simulink model "Switching_losses"  (R2015a)
settings: Solver=ode45  StartTime=0.0  StopTime=10.0  RelTol=1e-3
undefined symbols (not defined in the file): Vdc
settings Model: Creator=Caner  LastModifiedBy=Caner

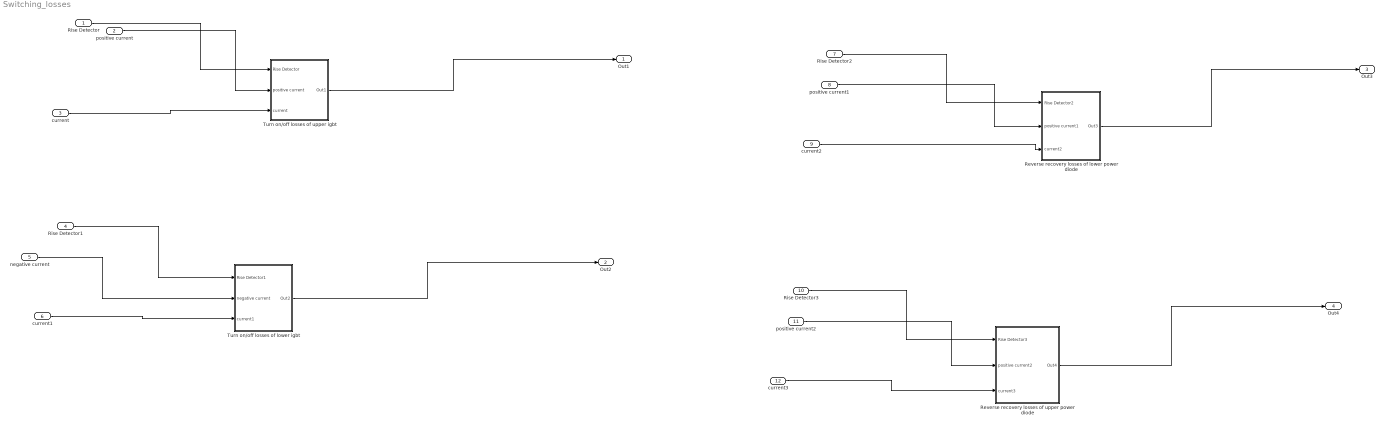
== system Switching_losses ==
  Rise Detector : Inport
  positive current : Inport  Port=2
  current : Inport  Port=3
  Rise Detector1 : Inport  Port=4
  negative current : Inport  Port=5
  current1 : Inport  Port=6
  Rise Detector2 : Inport  Port=7
  positive current1 : Inport  Port=8
  current2 : Inport  Port=9
  Rise Detector3 : Inport  Port=10
  positive current2 : Inport  Port=11
  current3 : Inport  Port=12
  "Reverse recovery losses of lower power diode " : Subsystem
  "Reverse recovery losses of upper power diode " : Subsystem
  "Turn on/off losses of lower igbt " : Subsystem
  "Turn on/off losses of upper igbt " : Subsystem
  Out1 : Outport
  Out2 : Outport  Port=2
  Out3 : Outport  Port=3
  Out4 : Outport  Port=4
  wires:
  Rise Detector/1 -> "Turn on/off losses of upper igbt "/1(Rise Detector)
  positive current/1 -> "Turn on/off losses of upper igbt "/2(positive current)
  current/1 -> "Turn on/off losses of upper igbt "/3(current)
  "Turn on/off losses of upper igbt "/1(Out1) -> Out1/1
  Rise Detector1/1 -> "Turn on/off losses of lower igbt "/1(Rise Detector1)
  negative current/1 -> "Turn on/off losses of lower igbt "/2(negative current)
  current1/1 -> "Turn on/off losses of lower igbt "/3(current1)
  "Turn on/off losses of lower igbt "/1(Out2) -> Out2/1
  Rise Detector2/1 -> "Reverse recovery losses of lower power diode "/1(Rise Detector2)
  positive current1/1 -> "Reverse recovery losses of lower power diode "/2(positive current1)
  current2/1 -> "Reverse recovery losses of lower power diode "/3(current2)
  "Reverse recovery losses of lower power diode "/1(Out3) -> Out3/1
  Rise Detector3/1 -> "Reverse recovery losses of upper power diode "/1(Rise Detector3)
  positive current2/1 -> "Reverse recovery losses of upper power diode "/2(positive current2)
  current3/1 -> "Reverse recovery losses of upper power diode "/3(current3)
  "Reverse recovery losses of upper power diode "/1(Out4) -> Out4/1

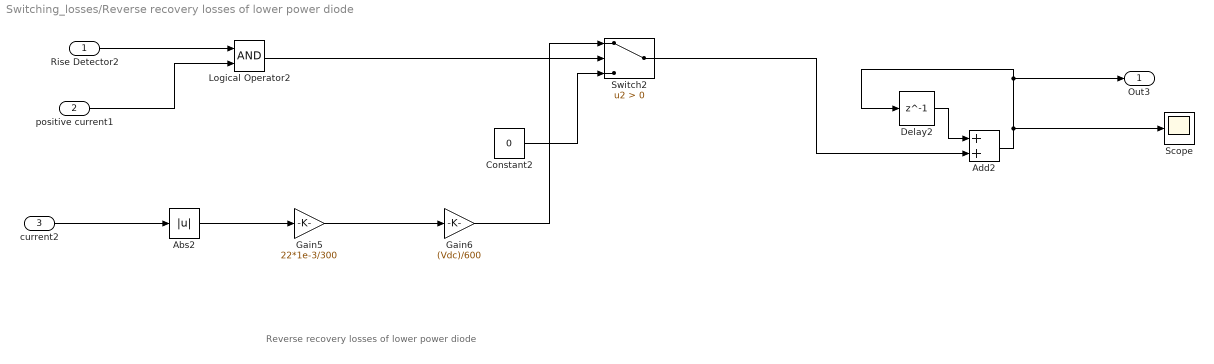
== system Switching_losses/Reverse recovery losses of lower power diode  ==
  note: Reverse recovery losses of lower power diode
  Rise Detector2 : Inport
  positive current1 : Inport  Port=2
  current2 : Inport  Port=3
  Abs2 : Abs
  Add2 : Sum
  Constant2 : Constant  Value=0
  Delay2 : Delay  DelayLength=1  InitialCondition=0
  Gain5 : Gain  Gain=22*1e-3/300
  Gain6 : Gain  Gain=(Vdc)/600
  Logical Operator2 : Logic  AllPortsSameDT=off  OutDataTypeStr=boolean
  Scope : Scope
  Switch2 : Switch  Criteria=u2 > Threshold
  Out3 : Outport
  wires:
  Gain5/1 -> Gain6/1
  Constant2/1 -> Switch2/3
  positive current1/1 -> Logical Operator2/2
  Add2/1 -> Scope/1, Out3/1, Delay2/1
  current2/1 -> Abs2/1
  Logical Operator2/1 -> Switch2/2
  Gain6/1 -> Switch2/1
  Rise Detector2/1 -> Logical Operator2/1
  Switch2/1 -> Add2/2
  Delay2/1 -> Add2/1
  Abs2/1 -> Gain5/1

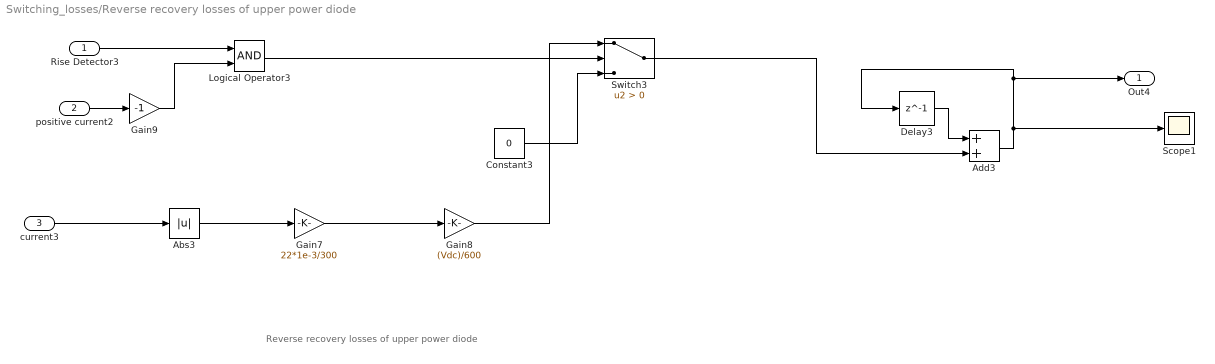
== system Switching_losses/Reverse recovery losses of upper power diode  ==
  note: Reverse recovery losses of upper power diode
  Rise Detector3 : Inport
  positive current2 : Inport  Port=2
  current3 : Inport  Port=3
  Abs3 : Abs
  Add3 : Sum
  Constant3 : Constant  Value=0
  Delay3 : Delay  DelayLength=1  InitialCondition=0
  Gain7 : Gain  Gain=22*1e-3/300
  Gain8 : Gain  Gain=(Vdc)/600
  Gain9 : Gain  Gain=-1
  Logical Operator3 : Logic  AllPortsSameDT=off  OutDataTypeStr=boolean
  Scope1 : Scope
  Switch3 : Switch  Criteria=u2 > Threshold
  Out4 : Outport
  wires:
  Abs3/1 -> Gain7/1
  Gain7/1 -> Gain8/1
  Gain8/1 -> Switch3/1
  Rise Detector3/1 -> Logical Operator3/1
  positive current2/1 -> Gain9/1
  Logical Operator3/1 -> Switch3/2
  current3/1 -> Abs3/1
  Add3/1 -> Scope1/1, Out4/1, Delay3/1
  Delay3/1 -> Add3/1
  Constant3/1 -> Switch3/3
  Gain9/1 -> Logical Operator3/2
  Switch3/1 -> Add3/2

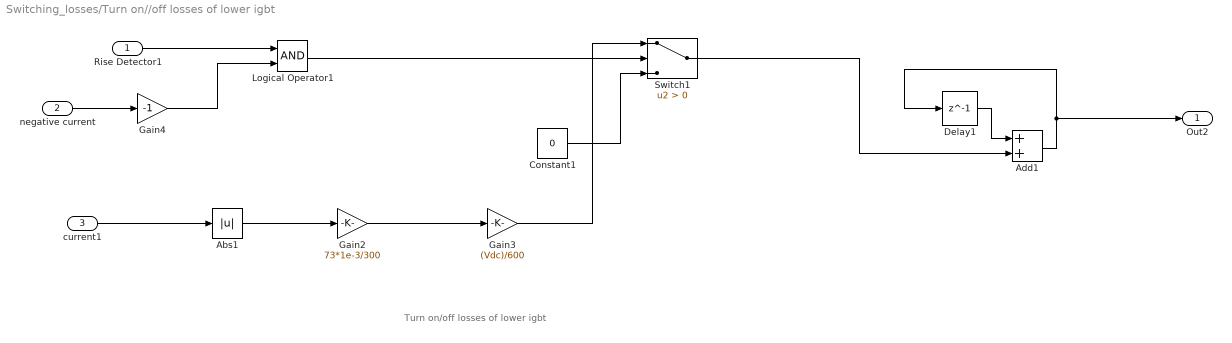
== system Switching_losses/Turn on//off losses of lower igbt  ==
  note: Turn on/off losses of lower igbt
  Rise Detector1 : Inport
  negative current : Inport  Port=2
  current1 : Inport  Port=3
  Abs1 : Abs
  Add1 : Sum
  Constant1 : Constant  Value=0
  Delay1 : Delay  DelayLength=1  InitialCondition=0
  Gain2 : Gain  Gain=73*1e-3/300
  Gain3 : Gain  Gain=(Vdc)/600
  Gain4 : Gain  Gain=-1
  Logical Operator1 : Logic  AllPortsSameDT=off  OutDataTypeStr=boolean
  Switch1 : Switch  Criteria=u2 > Threshold
  Out2 : Outport
  wires:
  Delay1/1 -> Add1/1
  current1/1 -> Abs1/1
  Gain3/1 -> Switch1/1
  Constant1/1 -> Switch1/3
  Gain4/1 -> Logical Operator1/2
  Logical Operator1/1 -> Switch1/2
  negative current/1 -> Gain4/1
  Rise Detector1/1 -> Logical Operator1/1
  Abs1/1 -> Gain2/1
  Add1/1 -> Out2/1, Delay1/1
  Gain2/1 -> Gain3/1
  Switch1/1 -> Add1/2

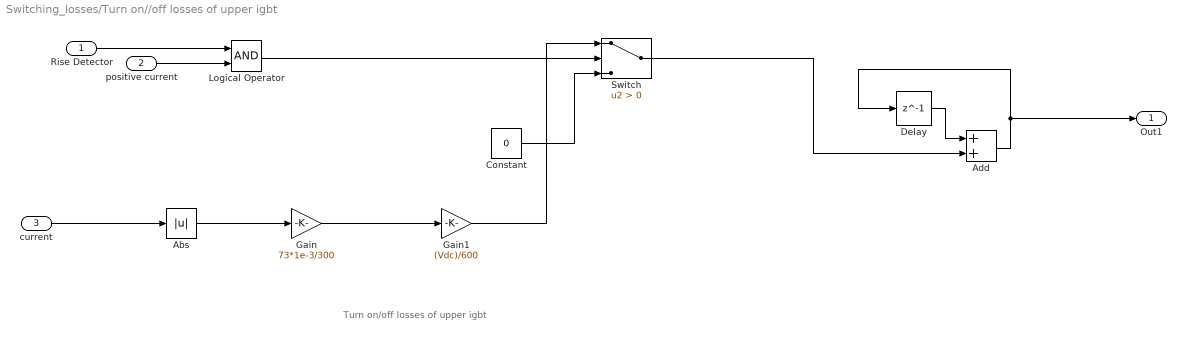
== system Switching_losses/Turn on//off losses of upper igbt  ==
  note: Turn on/off losses of upper igbt
  Rise Detector : Inport
  positive current : Inport  Port=2
  current : Inport  Port=3
  Abs : Abs
  Add : Sum
  Constant : Constant  Value=0
  Delay : Delay  DelayLength=1  InitialCondition=0
  Gain : Gain  Gain=73*1e-3/300
  Gain1 : Gain  Gain=(Vdc)/600
  Logical Operator : Logic  AllPortsSameDT=off  OutDataTypeStr=boolean
  Switch : Switch  Criteria=u2 > Threshold
  Out1 : Outport
  wires:
  Add/1 -> Out1/1, Delay/1
  Logical Operator/1 -> Switch/2
  current/1 -> Abs/1
  Abs/1 -> Gain/1
  Rise Detector/1 -> Logical Operator/1
  positive current/1 -> Logical Operator/2
  Gain/1 -> Gain1/1
  Gain1/1 -> Switch/1
  Constant/1 -> Switch/3
  Delay/1 -> Add/1
  Switch/1 -> Add/2
